simulink model "Dnote3lv3rd"  (R2016b)
settings: Solver=FixedStepDiscrete  StartTime=0.0  StopTime=simtime  RelTol=1e-3  EnableMultiTasking=on
PreLoadFcn:
  | simtime=0.0034;
undefined symbols (not defined in the file): Amp, fdesignblkfcn, Fin, Fs, FSC, gcbh, N, p, sw1, Ts
libraries: simulink x153, dspsnks4 x2, dspfdesign x1, dspvision x1, dsparch4 x1, dspmlti4 x1
(part 1 of 3)
settings Model: Creator=fumiaki  LastModifiedBy=l1tmn_main
settings Model: ModifiedComment=|
  | YUKI -- Sun Oct 02 16:05:03 2016 -- Version 1.144
  | シミュレーション前保存
settings Model: ModifiedHistory=|
  | YUKI -- Sun Oct 02 16:05:03 2016 -- Version 1.144
  | シミュレーション前保存
settings DataIOCC: LimitDataPoints=on  SaveFormat=Array  ReturnWorkspaceOutputsName=outn
settings OptimizationCC: ExpressionDepthLimit=2147483647  LifeSpan=inf
settings DebuggingCC: UnderspecifiedInitializationDetection=Classic  MergeDetectMultiDrivingBlocksExec=none  AllowSymbolicDim=off  StateNameClashWarn=warning  SFUnexpectedBacktrackingDiag=warning  SFNoUnconditionalDefaultTransitionDiag=warning  SFExecutionAtInitializationDiag=none
settings HardwareCC: ProdBitPerPointer=32  ProdBitPerSizeT=32  ProdBitPerPtrDiffT=32  ProdLargestAtomicFloat=None  ProdIntDivRoundTo=Undefined  ProdEndianess=Unspecified  ProdWordSize=32  ProdHWDeviceType=32-bit Generic
settings ModelReferenceCC: PropagateSignalLabelsOutOfModel=off
settings GRTTargetCC: TargetLangStandard=C89/C90 (ANSI)  GeneratePreprocessorConditionals=Disable all
settings ConfigComp: CovMetricSettings=dw  CovHtmlReporting=on  CovSaveCumulativeToWorkspaceVar=on  CovSaveSingleToWorkspaceVar=on  CovExternalEMLEnable=off  CovSFcnEnable=off

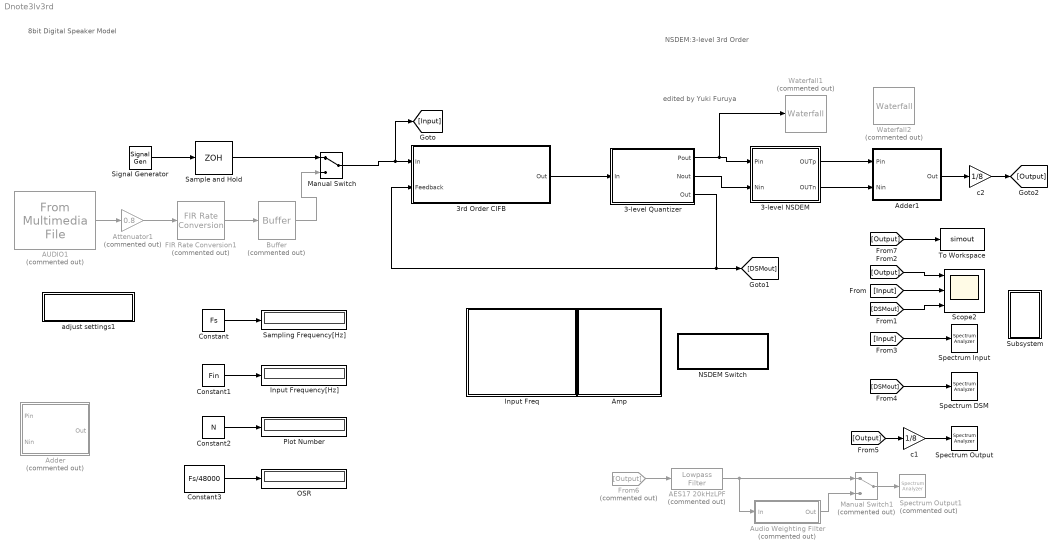
== system Dnote3lv3rd ==
  note: 8bit Digital Speaker Model
  note: edited by Yuki Furuya
  note: NSDEM:3-level 3rd Order
  "3-level NSDEM " : Subsystem  mask(3値化NSDEM){gain=[1 8 128], satulation=400}
      mask prompts: gain "フィードバック係数[1段目 2段目 ３段目]"; satulation "飽和器の値"
      mask init:
      | A=gain(1);
      | B=gain(2);
      | C=gain(3);
      | 
      | ns_fb=0;
      | 
      | SAT=satulation;
  3-level Quantizer : Subsystem
  3rd Order CIFB : Subsystem  mask(3次ΔΣ変調器(CIFB)){model=簡易モデル, FBgain=[1 3 3], INgain=[1 0 0 0], INTEGgain=[1 1 1], RESOgain=0, sat=inf}
      mask prompts: model "モデル選択"; FBgain "量子化器からのフィードバック係数 [a1 a2 a3]"; INgain "変調器から積分器の入力の係数[b1 b2 b3 b4]"; INTEGgain "積分器間の係数[c1 c2 c3]"; RESOgain "共鳴器の係数[g1]"; sat "飽和器の値[sat]"
      mask help:
      | 3次ΔΣ変調器(CIFB)のパラメータ設定
      | 簡易モデルにはa1=1; a2=3; a3=3; b1=1; b2~b4=0; c1=c2=c3=1; g1=0;を採用しています
      | 詳細モデルで任意の値を入力することが可能です。
      |
      | 係数設計にはΔΣtool boxがおすすめです。
      | 参考URL="https://pub.maruzen.co.jp/book_magazine/support/analog_digital/AppedixB_j.pdf"
      mask init:
      | if model=='簡易モデル'
      |     a1=1; a2=3; a3=3;
      |     b1=1; b2=0; b3=0; b4=0;
      |     c1=1; c2=1; c3=1;
      |     g1=0;
      |     sat=inf;
      | end
      | 
      | a1=FBgain(1);
      | a2=FBgain(2);
      | a3=FBgain(3);
      | 
      | b1=INgain(1);
      | b2=INgain(2);
      | b3=INgain(3);
      | b4=INgain(4);
      | 
      | c1=INTEGgain(1);
      | c2=INTEGgain(2);
      | c3=INTEGgain(3);
      | 
      | g1=RESOgain;
      | 
      | sat=sat;
      mask Help:
      | 3次ΔΣ変調器(CIFB)システムです。
      | 係数設定が必要です
      mask TypeOptions model: 簡易モデル | 詳細モデル
      mask Callback model:
      | enab = get_param(gcb,'model');
      | 
      | if enab=='簡易モデル'
      |     set_param(gcb,'MaskEnables',{'on','off','off','off','off','off',});
      | else
      |     set_param(gcb,'MaskEnables',{'on','on','on','on','on','on',});
      | end
  AES17 20kHzLPF : dspfdesign/Lowpass Filter  Commented=on  FilterType=FIR  DesignForMinimumOrder=on  FilterOrder=50  PassbandFrequency=20e3  StopbandFrequency=24e3  PassbandRipple=0.1  StopbandAttenuation=60  InheritSampleRate=on  SampleRate=48e3  SimulateUsing=Interpreted execution  roundingMode=Floor  coeffsDataTypeStr=fixdt(1,16)
  AUDIO1 : dspvision/From Multimedia File  Commented=on  inputFilename=/AudioSample.wav  loop=on  numPlays=1  outputStreams=Audio only  videoDataType=single  audioDataType=double  inheritSampleTime=on  userDefinedSampleTime=1/30  noAudioOutput=off  isIntensityVideo=off  fourcc=RGB  colorVideoFormat=One multidimensional signal  outputEOF=off  dataOrg=Column-major  audioFrameSize=q  computeAudioFrameSize=off  outSamplingMode=Sample based
  Adder : Subsystem  Commented=on  mask(加算器){enableerr=on, errratio=40}
      mask prompts: enableerr "製造誤差あり"; errratio "ミスマッチ[%]"
      mask help:
      | OUTpとOUTnを加算するモジュールです。
      | 誤差ありの信号が必要な場合はチェックボックスをONにしてください。
      mask init:
      | if ~enableerr
      |     err=ones(1,8);
      | else
      |     err=ones(1,8);
      |     by=errratio*0.01;
      |     a=1-by;
      |     b=1+by;
      |     rng(0,'twister');
      |     r = (b-1).*rand(1,8)+a;
      |     for i = 1:8
      |         err(i)=r(i);
      |     end
      | end
      mask Callback enableerr:
      | % Use the dialog callback to set the
      | % enabling and visibility of parameters
      | 
      | % Get the value of the Enable Bias checkbox
      | % unchecked = 'off'
      | % checked = 'on'
      | enab = get_param(gcb,'enableerr');
      | 
      | % Set the 'MaskVisililities' property for each parameters
      | if strcmp(enab,'on')
      |     set_param(gcb,'MaskVisibilities',{'on','on'});
      | else
      |     set_param(gcb,'MaskVisibilities',{'on','off'});
      | end
      | 
      | % Note that the value of the bias is not handled here.
      | % See the Initialization tab
  Adder1 : Subsystem  mask(加算器){enableerr=on, errratio=1}
      mask prompts: enableerr "製造誤差あり"; errratio "ミスマッチ[%]"
      mask help:
      | OUTpとOUTnを加算するモジュールです。
      | 誤差ありの信号が必要な場合はチェックボックスをONにしてください。
      mask init: same as Dnote3lv3rd/Adder
      mask Callback enableerr:
      | % Use the dialog callback to set the
      | % enabling and visibility of parameters
      | 
      | % Get the value of the Enable Bias checkbox
      | % unchecked = 'off'
      | % checked = 'on'
      | enab = get_param(gcb,'enableerr');
      | 
      | % Set the 'MaskVisililities' property for each parameters
      | if strcmp(enab,'on')
      |     set_param(gcb,'MaskVisibilities',{'on','on'});
      | else
      |     set_param(gcb,'MaskVisibilities',{'on','off'});
      | end
      | 
      | % Note that the value of the bias is not handled here.
      | % See the Initialization tab
  Amp : Subsystem  DialogController=hmiCreateDDGDialog  IsWebBlock=on  mask(MWDashboardBlock){webBlockId=3851c67f-551c-41d9-8c95-25d9ea438bcf, webBlockType=continuousknob, ShowInLibBrowser=on, ShowInitialText=on, HMISrcModelName=Dnote3lv3rd}
      mask prompts: webBlockId "WebBlock Id"; webBlockType "WebBlock Type"; HMISrcModelName "Source Model"
      mask Help: helpview([docroot '/mapfiles/simulink.map'], 'hmi_knob')
      mask Display:
      | if strcmp(get_param(bdroot(gcb),'BlockDiagramType'), 'library')
      |     image([(matlabroot) '/toolbox/simulink/hmi/icons/ContinuousKnob.png']);
      | end
  Attenuator1 : Gain  Commented=on  Gain=0.8  OutDataTypeStr=Inherit: Same as input  ParamDataTypeStr=Inherit: Same as input
  Audio Weighting Filter : Subsystem  Commented=on  DialogController=fdesignblkfcn  InitFcn=fdesignblkfcn(gcbh, {'InitFcn'});  mask(Audio Weighting Filter){}
      mask help: Design an audio weighting filter
      settings: CopyFcn=fdesignblkfcn(gcbh, {'CopyFcn'});
      mask Help: helpview(mapfilelocation('dsp'), 'dspaudioweightingfilter');
      mask Display: disp('Audio Weighting')
  Buffer : Buffer  Commented=on  N=1
  Constant : Constant  Value=Fs
  Constant1 : Constant  Value=Fin
  Constant2 : Constant  Value=N
  Constant3 : Constant  Value=Fs/48000
      mask Display: disp('OSR')
  FIR Rate Conversion1 : dspmlti4/FIR Rate Conversion  Commented=on  FilterSource=Dialog parameters  L=p  h=firpm(70,[0 .28 .32 1],[1 1 0 0])  M=q  FilterObject=Hm_firsrc  roundingMode=Floor  overflowMode=off  firstCoeffDataTypeStr=Inherit: Same word length as input  firstCoeffMin=[]  firstCoeffMax=[]  firstCoeffLastDataTypeStr=Inherit: Same word length as input  outputDataTypeStr=Inherit: Same as accumulator  outputMin=[]  outputMax=[]  outputLastDataTypeStr=Inherit: Same as accumulator
  From6 : From  Commented=on  GotoTag=Output
  Input Freq : Subsystem  DialogController=hmiCreateDDGDialog  IsWebBlock=on  mask(MWDashboardBlock){webBlockId=c57420c8-b641-4940-bc6c-5212ea864b9b, webBlockType=continuousknob, ShowInLibBrowser=on, ShowInitialText=on, HMISrcModelName=Dnote3lv3rd}
      mask prompts: webBlockId "WebBlock Id"; webBlockType "WebBlock Type"; HMISrcModelName "Source Model"
      mask Help: helpview([docroot '/mapfiles/simulink.map'], 'hmi_knob')
      mask Display:
      | if strcmp(get_param(bdroot(gcb),'BlockDiagramType'), 'library')
      |     image([(matlabroot) '/toolbox/simulink/hmi/icons/ContinuousKnob.png']);
      | end
  Input Frequency[Hz] : Display
  Manual Switch : ManualSwitch
  Manual Switch1 : ManualSwitch  Commented=on
  NSDEM Switch : Subsystem  DialogController=hmiCreateDDGDialog  IsWebBlock=on  mask(MathWorksWebBlock){webBlockId=b2297bbe-88b1-438d-afef-1205d982b626, webBlockType=sliderswitch, ShowInLibBrowser=on, ShowInitialText=on, HMISrcModelName=Dnote3lv3rd}
      mask prompts: webBlockId "WebBlock Id"; webBlockType "WebBlock Type"; HMISrcModelName "Source Model"
      mask Help: helpview([docroot '/mapfiles/simulink.map'], 'hmi_slider_switch')
      mask Display:
      | if strcmp(get_param(bdroot(gcb),'BlockDiagramType'), 'library')
      |     image([(matlabroot) '/toolbox/simulink/hmi/icons/SliderSwitch.png']);
      | end
  OSR : Display
  Plot Number : Display
  Sample and Hold : ZeroOrderHold  SampleTime=Ts
  Sampling Frequency[Hz] : Display
  Scope2 : Scope  NumInputPorts=3
  Signal Generator : SignalGenerator  Amplitude=Amp  Frequency=Fin
  Spectrum DSM : SpectrumAnalyzer
  Spectrum Input : SpectrumAnalyzer
  Spectrum Output : SpectrumAnalyzer
  Spectrum Output1 : SpectrumAnalyzer  Commented=on
  Subsystem : Subsystem
  To Workspace : ToWorkspace  VariableName=simout  SampleTime=-1
  Waterfall1 : dspsnks4/Waterfall  Commented=on  TraceProperties=off  NumTraces=8  CMapStr=red  TNewest=1  TOldest=0  HistoryLength=30  HistoryFull=Overwrite  UpdateInterval=1  ExportMode=Selected  MLExportName=ExportData  AutoExport=off  DisplayProperties=off  MouseMode=Orbit  AxisGrid=on  Snapshot=off  Suspend=off  SyncSnapshots=off  OpenScopeAtSimStart=off  FigPos=[657 331 413 324]  CameraView=[89.3889433100501 -276.781767245131 276.174253738902 0 5 3.5 0.767275197493131 1.68975903939443 -1.63514406758836 1.43035830301383 1 5 3]  InportDimsHint=[8 1]  AxisProperties=off  AxisColor='w'  XLabel=Speaker  YLabel=Logic  ZLabel=Time  TriggerProperties=off  TrigStartMode=Immediately  TrigStartT=0  TrigStartN=0  TrigStartFcn=trigbegin  TrigStopMode=Never  TrigStopT=0.1  TrigStopN=1  TrigStopFcn=trigend  TrigRearmMode=Never  TrigRearmT=0  TrigRearmN=0  TrigRearmFcn=trigrearm  XformProperties=on  XformMode=None  XformFcn=abs  XformExpr=(u+1)/2
      settings: YMin=0  YMax=1
  Waterfall2 : dspsnks4/Waterfall  Commented=on  TraceProperties=off  NumTraces=8  CMapStr=red  TNewest=1  TOldest=0  HistoryLength=30  HistoryFull=Overwrite  UpdateInterval=1  ExportMode=Selected  MLExportName=ExportData  AutoExport=off  DisplayProperties=off  MouseMode=Orbit  AxisGrid=on  Snapshot=off  Suspend=off  SyncSnapshots=off  OpenScopeAtSimStart=off  FigPos=[657 331 413 324]  CameraView=[89.3889433100501 -276.781767245131 276.174253738902 0 5 3.5 0.767275197493131 1.68975903939443 -1.63514406758836 1.43035830301383 1 5 3]  InportDimsHint=[8 1]  AxisProperties=off  AxisColor='w'  XLabel=Speaker  YLabel=Logic  ZLabel=Time  TriggerProperties=off  TrigStartMode=Immediately  TrigStartT=0  TrigStartN=0  TrigStartFcn=trigbegin  TrigStopMode=Never  TrigStopT=0.1  TrigStopN=1  TrigStopFcn=trigend  TrigRearmMode=Never  TrigRearmT=0  TrigRearmN=0  TrigRearmFcn=trigrearm  XformProperties=on  XformMode=None  XformFcn=abs  XformExpr=(u+1)/2
      settings: YMin=0  YMax=1
  adjust settings1 : Subsystem  Priority=1  mask(初期設定){N=48*128*50, Enablemode=on, EnableNSDEM=on, osr=128, Fin=1000, INGAIN=dBFS, Amp=0.5, AmpdB=-6}
      mask prompts: N "ポイント数(48*OSR*K, ※Kは任意の自然数)"; Enablemode "信号漏洩防止モード(推奨)"; EnableNSDEM "NSDEM使用"; osr "OSR(48kHz基準)"; Fin "入力周波数[Hz]"; INGAIN "入力振幅"; Amp "ダイヤル"; AmpdB "フルスケールに対する入力[dBFS]"
      mask help:
      | このモデルを動かすための初期設定です
      | 信号漏洩モードにチェックをいれると入力したポイント数にもっとも近い適切な値に変更してFFTを行う際に信号漏洩を防いでくれます。
      | 任意のポイント数を使用したい場合はチェックを入れないでください。
      |
      | NSDEM使用のチェックボックスはNSDEMを使用するか否かを選択することができます。
      mask init:
      | Fs=osr*48000; %サンプリング周波数
      | 
      | if EnableNSDEM
      |     sw=1;
      | else
      |     sw=0;
      | end
      | 
      | if INGAIN==1
      |     Amp=Amp;
      | else
      |     Amp=db2mag(AmpdB);
      | end
      | 
      | if Enablemode
      |      assignin('base', 'Noriginal', N);
      |     base = Fs/Fin;
      |     K = N/base;
      |     intK = round(K);
      |     N = base*intK;
      | end
      | 
      | 
      | [p,q] = rat(Fs/44100,0.0001) 
      | Ts=1/Fs;                                               %サンプリング周期
      | %fB = ceil(Fs*N/(2*osr));                   %帯域幅をfsの1/2*OSRと定義
      | %f0 = floor(2/3*fB);                            %入力信号を帯域幅内の2/3へ
      | %finrad= 2*pi/N*f0;                            %入力各周波数も正規化 to simlink
      | Offset = 1000;                                     %定常状態を扱うため初期動作の300plotは省く
      | simtime = (N+Offset)*Ts; 
      | %simtime = (N-1)*Ts; 
      | FSC=1;
      | 
      | %各変数をMATLABのワークスペースへ送る
      | assignin('base', 'simtime', simtime);
      | assignin('base','Fs' ,Fs);
      | assignin('base','Ts' ,Ts);
      | assignin('base','FSC' ,FSC);
      | assignin('base','Amp' ,Amp);
      | assignin('base','Fin' ,Fin);
      | assignin('base', 'simtime', simtime);
      | assignin('base', 'sw1', sw);
      | assignin('base', 'N', N);
      | assignin('base', 'Offset', Offset);
      | assignin('base', 'INGAIN',INGAIN );
      | assignin('base', 'p', p);
      | assignin('base', 'q', q);
      mask TypeOptions INGAIN: ダイヤル | dBFS
      mask Callback INGAIN:
      | enab = get_param(gcb,'INGAIN');
      | 
      | if enab=='ダイヤル'
      |     set_param(gcb,'MaskVisibilities',{'on','on','on','on','on','on','on','off'});
      | else
      |     set_param(gcb,'MaskVisibilities',{'on','on','on','on','on','on','off','on'});
      | end
      mask Display: disp('Simulation Settings')
  c1 : Gain  Gain=1/8  OutDataTypeStr=Inherit: Same as input  ParamDataTypeStr=Inherit: Same as input
  c2 : Gain  Gain=1/8  OutDataTypeStr=Inherit: Same as input  ParamDataTypeStr=Inherit: Same as input
  wires:
  3rd Order CIFB/1(Out) -> 3-level Quantizer/1(In)
  3-level Quantizer/3(Out) -> [DSMout], 3rd Order CIFB/2(Feedback)
  3-level Quantizer/1(Pout) -> Waterfall1/1, "3-level NSDEM "/1(Pin)
  Signal Generator/1 -> Sample and Hold/1
  AUDIO1/1 -> Attenuator1/1
  Attenuator1/1 -> FIR Rate Conversion1/1
  Sample and Hold/1 -> Manual Switch/1
  FIR Rate Conversion1/1 -> Buffer/1
  Manual Switch/1 -> [Input], 3rd Order CIFB/1(In)
  Buffer/1 -> Manual Switch/2
  Constant/1 -> Sampling Frequency[Hz]/1
  Constant1/1 -> Input Frequency[Hz]/1
  [Output] -> Scope2/1
  [Input] -> Scope2/2
  [DSMout] -> Scope2/3
  [Input] -> Spectrum Input/1
  [DSMout] -> Spectrum DSM/1
  From6/1 -> AES17 20kHzLPF/1
  Manual Switch1/1 -> Spectrum Output1/1
  AES17 20kHzLPF/1 -> Audio Weighting Filter/1(In), Manual Switch1/1
  Audio Weighting Filter/1(Out) -> Manual Switch1/2
  3-level Quantizer/2(Nout) -> "3-level NSDEM "/2(Nin)
  "3-level NSDEM "/1(OUTp) -> Adder1/1(Pin)
  "3-level NSDEM "/2(OUTn) -> Adder1/2(Nin)
  [Output] -> c1/1
  c1/1 -> Spectrum Output/1
  [Output] -> To Workspace/1
  c2/1 -> [Output]
  Adder1/1(Out) -> c2/1
  Constant2/1 -> Plot Number/1
  Constant3/1 -> OSR/1

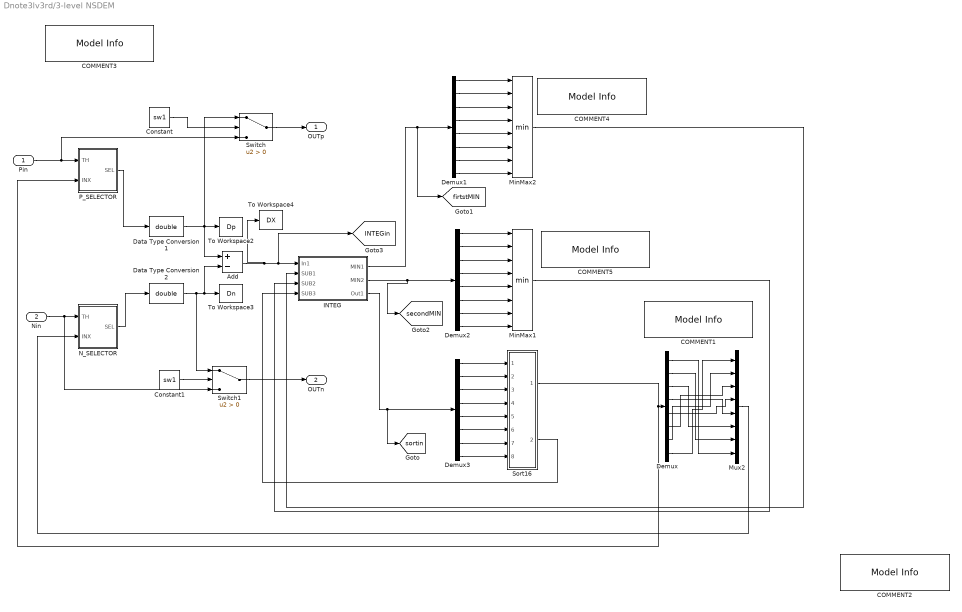
== system Dnote3lv3rd/3-level NSDEM  ==
  Pin : Inport
  Nin : Inport  Port=2
  Add : Sum  Inputs=+-
  COMMENT1 : simulink/Model-Wide Utilities/Model Info  Frame=on  DisplayStringWithTags=|  HorizontalTextAlignment=Center  LeftAlignmentValue=0.5  SourceBlockDiagram=Dnote  TagMaxNumber=20
      | バイトニックマージソートにより
      | スピーカの+側の使用頻度順に
      | 並び替え
  COMMENT2 : simulink/Model-Wide Utilities/Model Info  Frame=on  DisplayStringWithTags=p用に-側の使用頻度が少ない順に 並び替え  HorizontalTextAlignment=Center  LeftAlignmentValue=0.5  SourceBlockDiagram=Dnote  TagMaxNumber=20
  COMMENT3 : simulink/Model-Wide Utilities/Model Info  Frame=on  DisplayStringWithTags=どのスピーカを使用すべきか選択  HorizontalTextAlignment=Center  LeftAlignmentValue=0.5  SourceBlockDiagram=Dnote  TagMaxNumber=20
  COMMENT4 : simulink/Model-Wide Utilities/Model Info  Frame=on  DisplayStringWithTags=1段目の積分値の最小値  HorizontalTextAlignment=Center  LeftAlignmentValue=0.5  SourceBlockDiagram=Dnote  TagMaxNumber=20
  COMMENT5 : simulink/Model-Wide Utilities/Model Info  Frame=on  DisplayStringWithTags=2段目の積分値の最小値  HorizontalTextAlignment=Center  LeftAlignmentValue=0.5  SourceBlockDiagram=Dnote  TagMaxNumber=20
  Constant : Constant  Value=sw1
  Constant1 : Constant  Value=sw1
  Data Type Conversion1 : DataTypeConversion  OutDataTypeStr=double
  Data Type Conversion2 : DataTypeConversion  OutDataTypeStr=double
  Demux{,1..3} (4 alike) : Demux  Outputs=8
  INTEG : Subsystem
  MinMax1 : MinMax  Inputs=8
  MinMax2 : MinMax  Inputs=8
  Mux2 : Mux  Inputs=8
  N_SELECTOR : Subsystem
  P_SELECTOR : Subsystem
  Sort16 : Subsystem
  Switch : Switch  Criteria=u2 > Threshold
  Switch1 : Switch  Criteria=u2 > Threshold
  To Workspace2 : ToWorkspace  VariableName=Dp  SampleTime=-1
  To Workspace3 : ToWorkspace  VariableName=Dn  SampleTime=-1
  To Workspace4 : ToWorkspace  VariableName=DX  SampleTime=-1
  OUTp : Outport
  OUTn : Outport  Port=2
  tag scope: INTEGin=global, firtstMIN=global, secondMIN=global, sortin=global
  wires:
  Pin/1 -> Switch/3, P_SELECTOR/1(TH)
  P_SELECTOR/1(SEL) -> Data Type Conversion1/1
  Demux/8 -> Mux2/1
  Sort16/1(IDX) -> P_SELECTOR/2(INX), Demux/1
  Demux1/1 -> MinMax2/1
  Demux1/2 -> MinMax2/2
  Demux1/3 -> MinMax2/3
  Demux1/4 -> MinMax2/4
  Demux1/5 -> MinMax2/5
  Demux1/6 -> MinMax2/6
  Demux1/7 -> MinMax2/7
  Demux1/8 -> MinMax2/8
  Demux2/1 -> MinMax1/1
  Demux2/2 -> MinMax1/2
  Demux2/3 -> MinMax1/3
  Demux2/4 -> MinMax1/4
  Demux2/5 -> MinMax1/5
  Demux2/6 -> MinMax1/6
  Demux2/7 -> MinMax1/7
  Demux2/8 -> MinMax1/8
  N_SELECTOR/1(SEL) -> Data Type Conversion2/1
  Data Type Conversion1/1 -> To Workspace2/1, Switch/1, Add/1
  Add/1 -> To Workspace4/1, [INTEGin], INTEG/1(In1)
  INTEG/1(MIN1) -> [firtstMIN], Demux1/1
  INTEG/2(MIN2) -> [secondMIN], Demux2/1
  INTEG/3(Out1) -> [sortin], Demux3/1
  Demux3/1 -> Sort16/1(IN0)
  Demux3/2 -> Sort16/2(IN1)
  Demux3/3 -> Sort16/3(IN2)
  Demux3/4 -> Sort16/4(IN3)
  Demux3/5 -> Sort16/5(IN4)
  Demux3/6 -> Sort16/6(IN5)
  Demux3/7 -> Sort16/7(IN6)
  Demux3/8 -> Sort16/8(IN7)
  Sort16/2(MIN) -> INTEG/4(SUB3)
  MinMax2/1 -> INTEG/2(SUB1)
  MinMax1/1 -> INTEG/3(SUB2)
  Nin/1 -> Switch1/3, N_SELECTOR/1(TH)
  Mux2/1 -> N_SELECTOR/2(INX)
  Data Type Conversion2/1 -> Add/2, To Workspace3/1, Switch1/1
  Demux/7 -> Mux2/2
  Demux/2 -> Mux2/7
  Demux/1 -> Mux2/8
  Demux/3 -> Mux2/6
  Demux/6 -> Mux2/3
  Demux/4 -> Mux2/5
  Demux/5 -> Mux2/4
  Switch/1 -> OUTp/1
  Constant/1 -> Switch/2
  Switch1/1 -> OUTn/1
  Constant1/1 -> Switch1/2

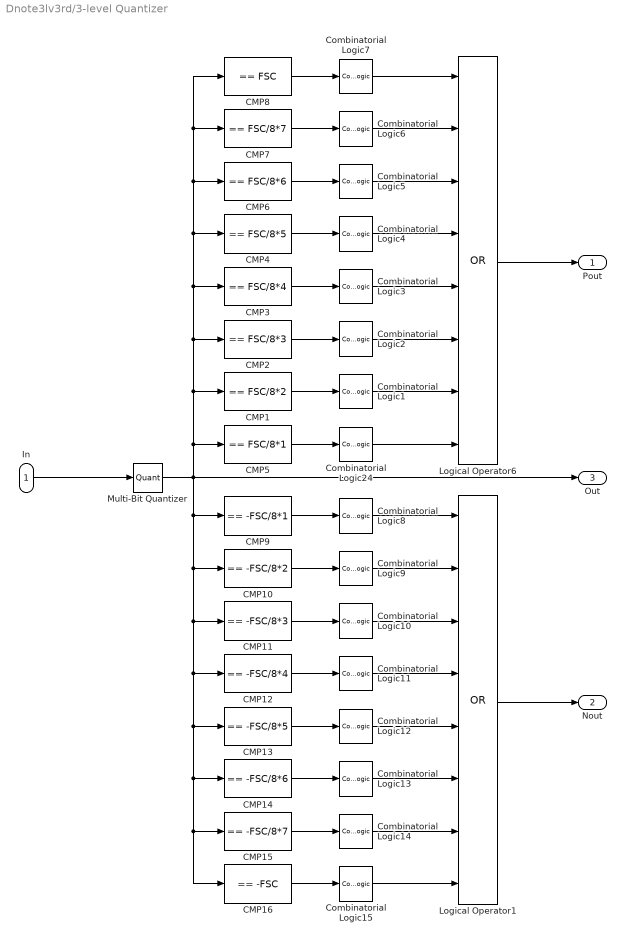
== system Dnote3lv3rd/3-level Quantizer ==
  In : Inport
  CMP1 : simulink/Logic and Bit Operations/Compare To Constant  relop===  const=FSC/8*2  OutDataTypeStr=boolean  ZeroCross=off
  CMP10 : simulink/Logic and Bit Operations/Compare To Constant  relop===  const=-FSC/8*2  OutDataTypeStr=boolean  ZeroCross=off
  CMP11 : simulink/Logic and Bit Operations/Compare To Constant  relop===  const=-FSC/8*3  OutDataTypeStr=boolean  ZeroCross=off
  CMP12 : simulink/Logic and Bit Operations/Compare To Constant  relop===  const=-FSC/8*4  OutDataTypeStr=boolean  ZeroCross=off
  CMP13 : simulink/Logic and Bit Operations/Compare To Constant  relop===  const=-FSC/8*5  OutDataTypeStr=boolean  ZeroCross=off
  CMP14 : simulink/Logic and Bit Operations/Compare To Constant  relop===  const=-FSC/8*6  OutDataTypeStr=boolean  ZeroCross=off
  CMP15 : simulink/Logic and Bit Operations/Compare To Constant  relop===  const=-FSC/8*7  OutDataTypeStr=boolean  ZeroCross=off
  CMP16 : simulink/Logic and Bit Operations/Compare To Constant  relop===  const=-FSC  OutDataTypeStr=boolean  ZeroCross=off
  CMP2 : simulink/Logic and Bit Operations/Compare To Constant  relop===  const=FSC/8*3  OutDataTypeStr=boolean  ZeroCross=off
  CMP3 : simulink/Logic and Bit Operations/Compare To Constant  relop===  const=FSC/8*4  OutDataTypeStr=boolean  ZeroCross=off
  CMP4 : simulink/Logic and Bit Operations/Compare To Constant  relop===  const=FSC/8*5  OutDataTypeStr=boolean  ZeroCross=off
  CMP5 : simulink/Logic and Bit Operations/Compare To Constant  relop===  const=FSC/8*1  OutDataTypeStr=boolean  ZeroCross=off
  CMP6 : simulink/Logic and Bit Operations/Compare To Constant  relop===  const=FSC/8*6  OutDataTypeStr=boolean  ZeroCross=off
  CMP7 : simulink/Logic and Bit Operations/Compare To Constant  relop===  const=FSC/8*7  OutDataTypeStr=boolean  ZeroCross=off
  CMP8 : simulink/Logic and Bit Operations/Compare To Constant  relop===  const=FSC  OutDataTypeStr=boolean  ZeroCross=off
  CMP9 : simulink/Logic and Bit Operations/Compare To Constant  relop===  const=-FSC/8*1  OutDataTypeStr=boolean  ZeroCross=off
  Combinatorial Logic1 : CombinatorialLogic  TruthTable=[0 0 0 0 0 0 0 0;1 1 0 0 0 0 0 0]
  Combinatorial Logic10 : CombinatorialLogic  TruthTable=[0 0 0 0 0 0 0 0;1 1 1 0 0 0 0 0]
  Combinatorial Logic11 : CombinatorialLogic  TruthTable=[0 0 0 0 0 0 0 0;1 1 1 1 0 0 0 0]
  Combinatorial Logic12 : CombinatorialLogic  TruthTable=[0 0 0 0 0 0 0 0;1 1 1 1 1 0 0 0]
  Combinatorial Logic13 : CombinatorialLogic  TruthTable=[0 0 0 0 0 0 0 0;1 1 1 1 1 1 0 0]
  Combinatorial Logic14 : CombinatorialLogic  TruthTable=[0 0 0 0 0 0 0 0;1 1 1 1 1 1 1 0]
  Combinatorial Logic15 : CombinatorialLogic  TruthTable=[0 0 0 0 0 0 0 0;1 1 1 1 1 1 1 1]
  Combinatorial Logic2 : CombinatorialLogic  TruthTable=[0 0 0 0 0 0 0 0;1 1 1 0 0 0 0 0]
  Combinatorial Logic24 : CombinatorialLogic  TruthTable=[0 0 0 0 0 0 0 0;1 0 0 0 0 0 0 0]
  Combinatorial Logic3 : CombinatorialLogic  TruthTable=[0 0 0 0 0 0 0 0;1 1 1 1 0 0 0 0]
  Combinatorial Logic4 : CombinatorialLogic  TruthTable=[0 0 0 0 0 0 0 0;1 1 1 1 1 0 0 0]
  Combinatorial Logic5 : CombinatorialLogic  TruthTable=[0 0 0 0 0 0 0 0;1 1 1 1 1 1 0 0]
  Combinatorial Logic6 : CombinatorialLogic  TruthTable=[0 0 0 0 0 0 0 0;1 1 1 1 1 1 1 0]
  Combinatorial Logic7 : CombinatorialLogic  TruthTable=[0 0 0 0 0 0 0 0;1 1 1 1 1 1 1 1]
  Combinatorial Logic8 : CombinatorialLogic  TruthTable=[0 0 0 0 0 0 0 0;1 0 0 0 0 0 0 0]
  Combinatorial Logic9 : CombinatorialLogic  TruthTable=[0 0 0 0 0 0 0 0;1 1 0 0 0 0 0 0]
  Logical Operator1 : Logic  Operator=OR  Inputs=8  AllPortsSameDT=off  OutDataTypeStr=boolean
  Logical Operator6 : Logic  Operator=OR  Inputs=8  AllPortsSameDT=off  OutDataTypeStr=boolean
  Multi-Bit Quantizer : Quantizer  QuantizationInterval=FSC/8
  Pout : Outport
  Nout : Outport  Port=2
  Out : Outport  Port=3
  wires:
  Multi-Bit Quantizer/1 -> CMP16/1, CMP15/1, CMP14/1, CMP13/1, CMP12/1, CMP11/1, CMP10/1, CMP9/1, Out/1, CMP8/1, CMP7/1, CMP6/1, CMP4/1, CMP3/1, CMP2/1, CMP1/1, CMP5/1
  Logical Operator6/1 -> Pout/1
  Logical Operator1/1 -> Nout/1
  CMP5/1 -> Combinatorial Logic24/1
  Combinatorial Logic24/1 -> Logical Operator6/8
  CMP1/1 -> Combinatorial Logic1/1
  Combinatorial Logic1/1 -> Logical Operator6/7
  CMP2/1 -> Combinatorial Logic2/1
  Combinatorial Logic2/1 -> Logical Operator6/6
  CMP3/1 -> Combinatorial Logic3/1
  Combinatorial Logic3/1 -> Logical Operator6/5
  CMP4/1 -> Combinatorial Logic4/1
  Combinatorial Logic4/1 -> Logical Operator6/4
  CMP6/1 -> Combinatorial Logic5/1
  Combinatorial Logic5/1 -> Logical Operator6/3
  CMP7/1 -> Combinatorial Logic6/1
  Combinatorial Logic6/1 -> Logical Operator6/2
  CMP8/1 -> Combinatorial Logic7/1
  Combinatorial Logic7/1 -> Logical Operator6/1
  CMP9/1 -> Combinatorial Logic8/1
  Combinatorial Logic8/1 -> Logical Operator1/1
  CMP10/1 -> Combinatorial Logic9/1
  Combinatorial Logic9/1 -> Logical Operator1/2
  CMP11/1 -> Combinatorial Logic10/1
  Combinatorial Logic10/1 -> Logical Operator1/3
  CMP12/1 -> Combinatorial Logic11/1
  Combinatorial Logic11/1 -> Logical Operator1/4
  CMP13/1 -> Combinatorial Logic12/1
  Combinatorial Logic12/1 -> Logical Operator1/5
  CMP14/1 -> Combinatorial Logic13/1
  Combinatorial Logic13/1 -> Logical Operator1/6
  CMP15/1 -> Combinatorial Logic14/1
  Combinatorial Logic14/1 -> Logical Operator1/7
  CMP16/1 -> Combinatorial Logic15/1
  Combinatorial Logic15/1 -> Logical Operator1/8
  In/1 -> Multi-Bit Quantizer/1

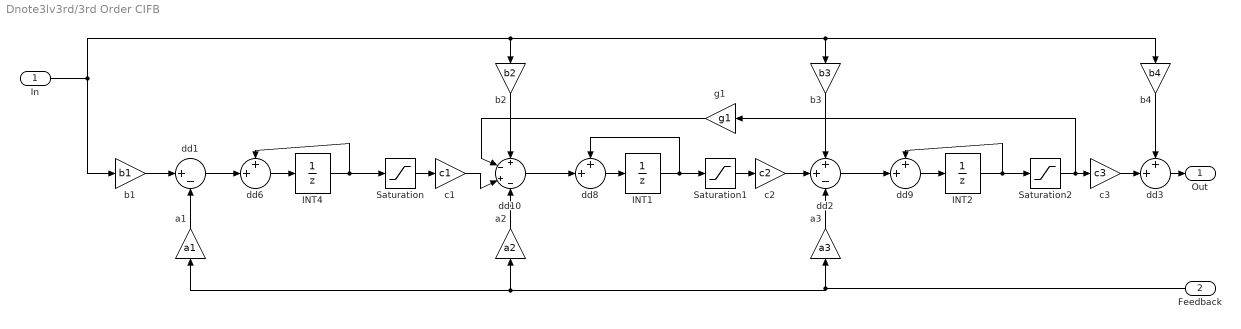
== system Dnote3lv3rd/3rd Order CIFB ==
  In : Inport
  Feedback : Inport  Port=2
  INT1 : UnitDelay  SampleTime=Ts
  INT2 : UnitDelay  SampleTime=Ts
  INT4 : UnitDelay  SampleTime=Ts
  Saturation : Saturate  UpperLimit=sat  LowerLimit=-sat
  Saturation1 : Saturate  UpperLimit=sat  LowerLimit=-sat
  Saturation2 : Saturate  UpperLimit=sat  LowerLimit=-sat
  a1 : Gain  Gain=a1  SampleTime=Ts  OutDataTypeStr=Inherit: Same as input  ParamDataTypeStr=Inherit: Same as input
  a2 : Gain  Gain=a2  SampleTime=Ts  OutDataTypeStr=Inherit: Same as input  ParamDataTypeStr=Inherit: Same as input
  a3 : Gain  Gain=a3  SampleTime=Ts  OutDataTypeStr=Inherit: Same as input  ParamDataTypeStr=Inherit: Same as input
  b1 : Gain  Gain=b1  SampleTime=Ts  SaturateOnIntegerOverflow=on  OutDataTypeStr=Inherit: Same as input  ParamDataTypeStr=Inherit: Same as input
  b2 : Gain  Gain=b2  SampleTime=Ts  SaturateOnIntegerOverflow=on  OutDataTypeStr=Inherit: Same as input  ParamDataTypeStr=Inherit: Same as input
  b3 : Gain  Gain=b3  SampleTime=Ts  SaturateOnIntegerOverflow=on  OutDataTypeStr=Inherit: Same as input  ParamDataTypeStr=Inherit: Same as input
  b4 : Gain  Gain=b4  SampleTime=Ts  SaturateOnIntegerOverflow=on  OutDataTypeStr=Inherit: Same as input  ParamDataTypeStr=Inherit: Same as input
  c1 : Gain  Gain=c1  SampleTime=Ts  OutDataTypeStr=Inherit: Same as input  ParamDataTypeStr=Inherit: Same as input
  c2 : Gain  Gain=c2  SampleTime=Ts  OutDataTypeStr=Inherit: Same as input  ParamDataTypeStr=Inherit: Same as input
  c3 : Gain  Gain=c3  SampleTime=Ts  OutDataTypeStr=Inherit: Same as input  ParamDataTypeStr=Inherit: Same as input
  dd1 : Sum  Inputs=|+-  OutDataTypeStr=double  SampleTime=Ts  SaturateOnIntegerOverflow=on  InputSameDT=on
  dd10 : Sum  Inputs=+-+-  OutDataTypeStr=double  SampleTime=Ts  SaturateOnIntegerOverflow=on  InputSameDT=on
  dd2 : Sum  Inputs=++-  OutDataTypeStr=double  SampleTime=Ts  SaturateOnIntegerOverflow=on  InputSameDT=on
  dd3 : Sum  Inputs=++|  OutDataTypeStr=double  SampleTime=Ts  SaturateOnIntegerOverflow=on  InputSameDT=on
  dd6 : Sum  Inputs=++|  OutDataTypeStr=double  SaturateOnIntegerOverflow=on  InputSameDT=on
  dd8 : Sum  Inputs=++|  OutDataTypeStr=double  SaturateOnIntegerOverflow=on  InputSameDT=on
  dd9 : Sum  Inputs=++|  OutDataTypeStr=double  SaturateOnIntegerOverflow=on  InputSameDT=on
  g1 : Gain  Gain=g1  SampleTime=Ts  SaturateOnIntegerOverflow=on  OutDataTypeStr=Inherit: Same as input  ParamDataTypeStr=Inherit: Same as input
  Out : Outport
  wires:
  dd1/1 -> dd6/2
  dd6/1 -> INT4/1
  dd8/1 -> INT1/1
  dd2/1 -> dd9/2
  dd9/1 -> INT2/1
  INT1/1 -> dd8/1, Saturation1/1
  a1/1 -> dd1/2
  INT2/1 -> dd9/1, Saturation2/1
  In/1 -> b4/1, b3/1, b2/1, b1/1
  INT4/1 -> dd6/1, Saturation/1
  Saturation/1 -> c1/1
  b1/1 -> dd1/1
  Saturation1/1 -> c2/1
  Saturation2/1 -> g1/1, c3/1
  Feedback/1 -> a2/1, a1/1, a3/1
  b2/1 -> dd10/1
  a3/1 -> dd2/3
  c2/1 -> dd2/2
  b3/1 -> dd2/1
  c3/1 -> dd3/2
  dd3/1 -> Out/1
  b4/1 -> dd3/1
  c1/1 -> dd10/3
  g1/1 -> dd10/2
  a2/1 -> dd10/4
  dd10/1 -> dd8/2

== system Dnote3lv3rd/Adder ==
  Pin : Inport
  Nin : Inport  Port=2
  Demux : Demux  Outputs=8
  Demux1 : Demux  Outputs=8
  c1 : Gain  Gain=err(1)  OutDataTypeStr=Inherit: Same as input  ParamDataTypeStr=Inherit: Same as input
  c2 : Gain  Gain=err(2)  OutDataTypeStr=Inherit: Same as input  ParamDataTypeStr=Inherit: Same as input
  c3 : Gain  Gain=err(3)  OutDataTypeStr=Inherit: Same as input  ParamDataTypeStr=Inherit: Same as input
  c4 : Gain  Gain=err(4)  OutDataTypeStr=Inherit: Same as input  ParamDataTypeStr=Inherit: Same as input
  c5 : Gain  Gain=err(5)  OutDataTypeStr=Inherit: Same as input  ParamDataTypeStr=Inherit: Same as input
  c6 : Gain  Gain=err(6)  OutDataTypeStr=Inherit: Same as input  ParamDataTypeStr=Inherit: Same as input
  c7 : Gain  Gain=err(7)  OutDataTypeStr=Inherit: Same as input  ParamDataTypeStr=Inherit: Same as input
  c8 : Gain  Gain=err(8)  OutDataTypeStr=Inherit: Same as input  ParamDataTypeStr=Inherit: Same as input
  dd{1..2,4..9} (8 alike) : Sum  Inputs=+-  OutDataTypeStr=double  SaturateOnIntegerOverflow=on  InputSameDT=on
  dd3 : Sum  Inputs=|++++++++  OutDataTypeStr=double  SaturateOnIntegerOverflow=on  InputSameDT=on
  Out : Outport
  wires:
  Pin/1 -> Demux/1
  dd3/1 -> Out/1
  Nin/1 -> Demux1/1
  Demux/1 -> dd1/1
  Demux1/8 -> dd1/2
  Demux/2 -> dd2/1
  Demux1/7 -> dd2/2
  Demux/3 -> dd4/1
  Demux1/6 -> dd4/2
  Demux/4 -> dd5/1
  Demux1/5 -> dd5/2
  Demux/5 -> dd6/1
  Demux1/4 -> dd6/2
  Demux/6 -> dd7/1
  Demux1/3 -> dd7/2
  Demux/7 -> dd9/1
  Demux1/2 -> dd9/2
  Demux/8 -> dd8/1
  Demux1/1 -> dd8/2
  dd1/1 -> c1/1
  c1/1 -> dd3/1
  dd2/1 -> c2/1
  c2/1 -> dd3/3
  dd4/1 -> c3/1
  c3/1 -> dd3/4
  dd5/1 -> c4/1
  c4/1 -> dd3/5
  dd6/1 -> c5/1
  c5/1 -> dd3/6
  dd7/1 -> c6/1
  c6/1 -> dd3/7
  dd9/1 -> c7/1
  c7/1 -> dd3/8
  dd8/1 -> c8/1
  c8/1 -> dd3/2

== system Dnote3lv3rd/Adder1 ==
  Pin : Inport
  Nin : Inport  Port=2
  Demux : Demux  Outputs=8
  Demux1 : Demux  Outputs=8
  c10 : Gain  Gain=err(6)  OutDataTypeStr=Inherit: Same as input  ParamDataTypeStr=Inherit: Same as input
  c11 : Gain  Gain=err(7)  OutDataTypeStr=Inherit: Same as input  ParamDataTypeStr=Inherit: Same as input
  c12 : Gain  Gain=err(8)  OutDataTypeStr=Inherit: Same as input  ParamDataTypeStr=Inherit: Same as input
  c13 : Gain  Gain=err(7)  OutDataTypeStr=Inherit: Same as input  ParamDataTypeStr=Inherit: Same as input
  c14 : Gain  Gain=err(8)  OutDataTypeStr=Inherit: Same as input  ParamDataTypeStr=Inherit: Same as input
  c15 : Gain  Gain=err(1)  OutDataTypeStr=Inherit: Same as input  ParamDataTypeStr=Inherit: Same as input
  c16 : Gain  Gain=err(2)  OutDataTypeStr=Inherit: Same as input  ParamDataTypeStr=Inherit: Same as input
  c17 : Gain  Gain=err(3)  OutDataTypeStr=Inherit: Same as input  ParamDataTypeStr=Inherit: Same as input
  c18 : Gain  Gain=err(4)  OutDataTypeStr=Inherit: Same as input  ParamDataTypeStr=Inherit: Same as input
  c19 : Gain  Gain=err(5)  OutDataTypeStr=Inherit: Same as input  ParamDataTypeStr=Inherit: Same as input
  c4 : Gain  Gain=err(6)  OutDataTypeStr=Inherit: Same as input  ParamDataTypeStr=Inherit: Same as input
  c5 : Gain  Gain=err(1)  OutDataTypeStr=Inherit: Same as input  ParamDataTypeStr=Inherit: Same as input
  c6 : Gain  Gain=err(2)  OutDataTypeStr=Inherit: Same as input  ParamDataTypeStr=Inherit: Same as input
  c7 : Gain  Gain=err(3)  OutDataTypeStr=Inherit: Same as input  ParamDataTypeStr=Inherit: Same as input
  c8 : Gain  Gain=err(4)  OutDataTypeStr=Inherit: Same as input  ParamDataTypeStr=Inherit: Same as input
  c9 : Gain  Gain=err(5)  OutDataTypeStr=Inherit: Same as input  ParamDataTypeStr=Inherit: Same as input
  dd3 : Sum  Inputs=|++++++++--------  OutDataTypeStr=double  SaturateOnIntegerOverflow=on  InputSameDT=on
  Out : Outport
  wires:
  c7/1 -> dd3/6
  c11/1 -> dd3/2
  Demux/2 -> c6/1
  Demux/3 -> c7/1
  Demux/6 -> c10/1
  c14/1 -> dd3/9
  c12/1 -> dd3/1
  c5/1 -> dd3/8
  c6/1 -> dd3/7
  Demux/4 -> c8/1
  c19/1 -> dd3/12
  c18/1 -> dd3/13
  c16/1 -> dd3/15
  Demux1/2 -> c16/1
  Demux/5 -> c9/1
  Demux/7 -> c11/1
  Demux/8 -> c12/1
  Demux/1 -> c5/1
  c9/1 -> dd3/4
  Demux1/3 -> c17/1
  Demux1/4 -> c18/1
  c4/1 -> dd3/11
  c10/1 -> dd3/3
  c8/1 -> dd3/5
  c13/1 -> dd3/10
  c15/1 -> dd3/16
  Demux1/6 -> c4/1
  Pin/1 -> Demux/1
  dd3/1 -> Out/1
  Demux1/7 -> c13/1
  Nin/1 -> Demux1/1
  Demux1/8 -> c14/1
  c17/1 -> dd3/14
  Demux1/1 -> c15/1
  Demux1/5 -> c19/1

== system Dnote3lv3rd/Amp ==

== system Dnote3lv3rd/Audio Weighting Filter ==
  In : Inport
  Generated Filter Block : dsparch4/Biquad Filter  Tag=BlockMethodSubSystem  IIRFiltStruct=Direct form II  CoeffSource=Specify via dialog  BiQuadCoeffs=[2.07591518974758993e-08 4.15183037949517986e-08 2.07591518974758993e-08 1 -1.97521362266648004 0.975367213791809906;1 -2 1 1 -1.99913562159154545 0.999135704628153154;1 -2 1 1 -1.99995786915622609 0.999957869599978122]  a0Flag=Warning  IC=0  ICnum=0  ICden=0  InputProcessing=Columns as channels (frame based)  denAccumFracLength=30  denProdOutputFracLength=30  secondMemoryFracLength=15  roundingMode=Floor  overflowMode=off  ScaleValues=[0.000153591125329866101;1;1;15153694.3885192499]  optimizeScaleValues=off  ScaleValueMode=Specify via input port (g)  scaleValueFracLength=14  FilterSource=Specify via dialog  FilterObject=BQF
  Out : Outport
  wires:
  In/1 -> Generated Filter Block/1
  Generated Filter Block/1 -> Out/1

== system Dnote3lv3rd/Input Freq ==

== system Dnote3lv3rd/NSDEM Switch ==

== system Dnote3lv3rd/Subsystem ==
  Demux{1..4} (4 alike) : Demux  Outputs=8
  Scope{,1..3} (4 alike) : Scope  NumInputPorts=8
  wires:
  [sortin] -> Demux3/1
  Demux3/1 -> Scope/1
  Demux3/2 -> Scope/2
  Demux3/3 -> Scope/3
  Demux3/4 -> Scope/4
  Demux3/5 -> Scope/5
  Demux3/6 -> Scope/6
  Demux3/7 -> Scope/7
  Demux3/8 -> Scope/8
  Demux1/1 -> Scope1/1
  Demux1/2 -> Scope1/2
  Demux1/3 -> Scope1/3
  Demux1/4 -> Scope1/4
  Demux1/5 -> Scope1/5
  Demux1/6 -> Scope1/6
  Demux1/7 -> Scope1/7
  Demux1/8 -> Scope1/8
  [secondMIN] -> Demux2/1
  Demux2/1 -> Scope2/1
  Demux2/2 -> Scope2/2
  Demux2/3 -> Scope2/3
  Demux2/4 -> Scope2/4
  Demux2/5 -> Scope2/5
  Demux2/6 -> Scope2/6
  Demux2/7 -> Scope2/7
  Demux2/8 -> Scope2/8
  [firtstMIN] -> Demux1/1
  [INTEGin] -> Demux4/1
  Demux4/1 -> Scope3/1
  Demux4/2 -> Scope3/2
  Demux4/3 -> Scope3/3
  Demux4/4 -> Scope3/4
  Demux4/5 -> Scope3/5
  Demux4/6 -> Scope3/6
  Demux4/7 -> Scope3/7
  Demux4/8 -> Scope3/8

== system Dnote3lv3rd/adjust settings1 ==
  note: This subsystem is empty.
      | It is used for setting parameter values (in the mask).

== system Dnote3lv3rd/3-level NSDEM /INTEG ==
  In1 : Inport
  SUB1 : Inport  Port=2
  SUB2 : Inport  Port=3
  SUB3 : Inport  Port=4
  COMMENT1 : simulink/Model-Wide Utilities/Model Info  Frame=on  DisplayStringWithTags=スピーカごとに使用回数を積分  HorizontalTextAlignment=Center  LeftAlignmentValue=0.5  SourceBlockDiagram=Dnote  TagMaxNumber=20
  COMMENT2 : simulink/Model-Wide Utilities/Model Info  Frame=on  DisplayStringWithTags=格段の積分値を引くことによって 積分値が飽和しないようにしている  HorizontalTextAlignment=Center  LeftAlignmentValue=0.5  SourceBlockDiagram=Dnote  TagMaxNumber=20
  Demux : Demux  Outputs=8
  INTEG4_1 : Subsystem
  INTEG4_2 : Subsystem
  INTEG4_3 : Subsystem
  INTEG4_4 : Subsystem
  INTEG4_5 : Subsystem
  INTEG4_6 : Subsystem
  INTEG4_7 : Subsystem
  INTEG4_8 : Subsystem
  Mux : Mux  Inputs=8
  Mux1 : Mux  Inputs=8
  Mux2 : Mux  Inputs=8
  MIN1 : Outport
  MIN2 : Outport  Port=2
  Out1 : Outport  Port=3
  wires:
  Demux/8 -> INTEG4_8/1(IN)
  Demux/7 -> INTEG4_7/1(IN)
  Demux/6 -> INTEG4_6/1(IN)
  Demux/5 -> INTEG4_5/1(IN)
  Demux/4 -> INTEG4_4/1(IN)
  Demux/3 -> INTEG4_3/1(IN)
  Demux/2 -> INTEG4_2/1(IN)
  Demux/1 -> INTEG4_1/1(IN)
  INTEG4_1/1(OUT1) -> Mux/1
  INTEG4_2/1(OUT1) -> Mux/2
  INTEG4_3/1(OUT1) -> Mux/3
  INTEG4_4/1(OUT1) -> Mux/4
  INTEG4_5/1(OUT1) -> Mux/5
  INTEG4_6/1(OUT1) -> Mux/6
  INTEG4_7/1(OUT1) -> Mux/7
  INTEG4_8/1(OUT1) -> Mux/8
  INTEG4_1/2(OUT2) -> Mux1/1
  INTEG4_2/2(OUT2) -> Mux1/2
  INTEG4_3/2(OUT2) -> Mux1/3
  INTEG4_4/2(OUT2) -> Mux1/4
  INTEG4_5/2(OUT2) -> Mux1/5
  INTEG4_6/2(OUT2) -> Mux1/6
  INTEG4_7/2(OUT2) -> Mux1/7
  INTEG4_8/2(OUT2) -> Mux1/8
  INTEG4_8/3(OUT3) -> Mux2/8
  INTEG4_7/3(OUT3) -> Mux2/7
  INTEG4_6/3(OUT3) -> Mux2/6
  INTEG4_5/3(OUT3) -> Mux2/5
  INTEG4_4/3(OUT3) -> Mux2/4
  INTEG4_3/3(OUT3) -> Mux2/3
  INTEG4_2/3(OUT3) -> Mux2/2
  INTEG4_1/3(OUT3) -> Mux2/1
  Mux/1 -> MIN1/1
  Mux1/1 -> MIN2/1
  Mux2/1 -> Out1/1
  In1/1 -> Demux/1
  SUB3/1 -> INTEG4_8/4(SUB3), INTEG4_7/4(SUB3), INTEG4_6/4(SUB3), INTEG4_5/4(SUB3), INTEG4_4/4(SUB3), INTEG4_3/4(SUB3), INTEG4_2/4(SUB3), INTEG4_1/4(SUB3)
  SUB2/1 -> INTEG4_8/3(SUB2), INTEG4_7/3(SUB2), INTEG4_6/3(SUB2), INTEG4_5/3(SUB2), INTEG4_4/3(SUB2), INTEG4_3/3(SUB2), INTEG4_2/3(SUB2), INTEG4_1/3(SUB2)
  SUB1/1 -> INTEG4_8/2(SUB1), INTEG4_7/2(SUB1), INTEG4_6/2(SUB1), INTEG4_5/2(SUB1), INTEG4_4/2(SUB1), INTEG4_3/2(SUB1), INTEG4_2/2(SUB1), INTEG4_1/2(SUB1)

== system Dnote3lv3rd/3-level NSDEM /N_SELECTOR ==
  TH : Inport
  INX : Inport  Port=2
  Constant : Constant  Value=[0 0 0 0 0 0 0 0]
  Demux : Demux  Outputs=8
  Demux1 : Demux  Outputs=8
  Logical Operator : Logic  Operator=OR  Inputs=8  AllPortsSameDT=off  OutDataTypeStr=boolean
  Subsystem : Subsystem
  Subsystem1 : Subsystem
  Subsystem2 : Subsystem
  Subsystem3 : Subsystem
  Subsystem4 : Subsystem
  Subsystem5 : Subsystem
  Subsystem6 : Subsystem
  Subsystem7 : Subsystem
  Switch{,1..7} (8 alike) : Switch  Criteria=u2 ~= 0
  SEL : Outport
  wires:
  Demux1/8 -> Switch7/2
  Demux1/7 -> Switch6/2
  Demux1/6 -> Switch5/2
  Demux1/5 -> Switch4/2
  Demux1/4 -> Switch3/2
  Demux1/3 -> Switch2/2
  Demux1/2 -> Switch1/2
  Subsystem/1(Out1) -> Switch/1
  Demux1/1 -> Switch/2
  Demux/1 -> Subsystem/1(In1)
  INX/1 -> Demux/1
  TH/1 -> Demux1/1
  Subsystem1/1(Out1) -> Switch1/1
  Subsystem2/1(Out1) -> Switch2/1
  Subsystem3/1(Out1) -> Switch3/1
  Subsystem4/1(Out1) -> Switch4/1
  Subsystem5/1(Out1) -> Switch5/1
  Subsystem6/1(Out1) -> Switch6/1
  Subsystem7/1(Out1) -> Switch7/1
  Demux/2 -> Subsystem1/1(In1)
  Demux/3 -> Subsystem2/1(In1)
  Demux/4 -> Subsystem3/1(In1)
  Demux/5 -> Subsystem4/1(In1)
  Demux/6 -> Subsystem5/1(In1)
  Demux/7 -> Subsystem6/1(In1)
  Demux/8 -> Subsystem7/1(In1)
  Switch/1 -> Logical Operator/1
  Switch1/1 -> Logical Operator/2
  Switch2/1 -> Logical Operator/3
  Switch3/1 -> Logical Operator/4
  Switch4/1 -> Logical Operator/5
  Switch5/1 -> Logical Operator/6
  Switch6/1 -> Logical Operator/7
  Switch7/1 -> Logical Operator/8
  Constant/1 -> Switch4/3, Switch/3, Switch1/3, Switch2/3, Switch3/3, Switch5/3, Switch6/3, Switch7/3
  Logical Operator/1 -> SEL/1

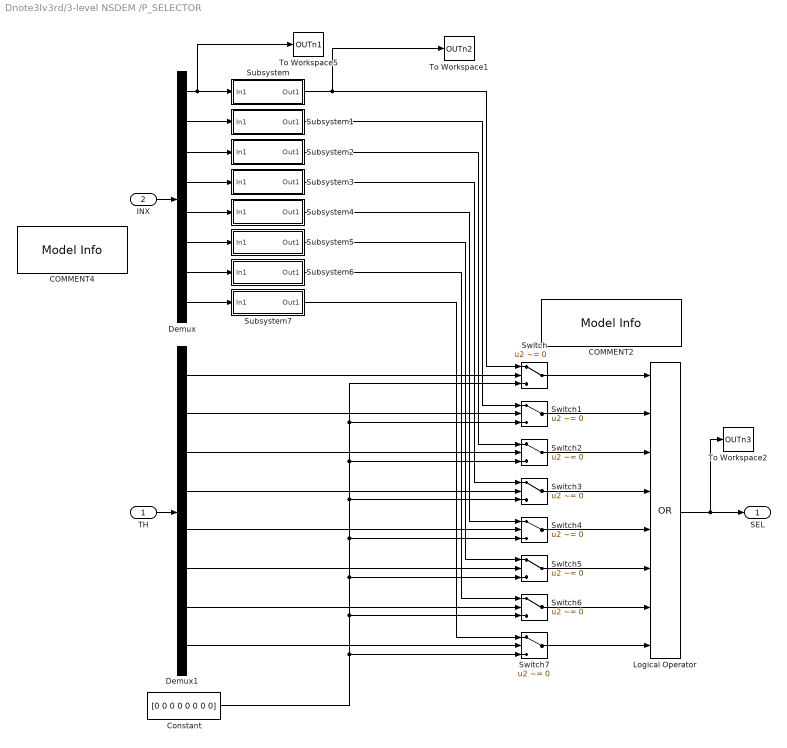
== system Dnote3lv3rd/3-level NSDEM /P_SELECTOR ==
  TH : Inport
  INX : Inport  Port=2
  COMMENT2 : simulink/Model-Wide Utilities/Model Info  Frame=on  DisplayStringWithTags=温度計コードによりスピーカの 使用個数分出力  HorizontalTextAlignment=Center  LeftAlignmentValue=0.5  SourceBlockDiagram=Dnote  TagMaxNumber=20
  COMMENT4 : simulink/Model-Wide Utilities/Model Info  Frame=on  DisplayStringWithTags=|  HorizontalTextAlignment=Center  LeftAlignmentValue=0.5  SourceBlockDiagram=Dnote  TagMaxNumber=20
      | スピーカの使用回数が少ない順に
      | 並び替えられて入力
      | 入力されるのは使用回数じゃなくどのスピーカが少ないのか
  Constant : Constant  Value=[0 0 0 0 0 0 0 0]
  Demux : Demux  Outputs=8
  Demux1 : Demux  Outputs=8
  Logical Operator : Logic  Operator=OR  Inputs=8  AllPortsSameDT=off  OutDataTypeStr=boolean
  Subsystem : Subsystem
  Subsystem1 : Subsystem
  Subsystem2 : Subsystem
  Subsystem3 : Subsystem
  Subsystem4 : Subsystem
  Subsystem5 : Subsystem
  Subsystem6 : Subsystem
  Subsystem7 : Subsystem
  Switch{,1..7} (8 alike) : Switch  Criteria=u2 ~= 0
  To Workspace1 : ToWorkspace  VariableName=OUTn2  SampleTime=-1
  To Workspace2 : ToWorkspace  VariableName=OUTn3  SampleTime=-1
  To Workspace5 : ToWorkspace  VariableName=OUTn1  SampleTime=-1
  SEL : Outport
  wires:
  Demux1/8 -> Switch7/2
  Demux1/7 -> Switch6/2
  Demux1/6 -> Switch5/2
  Demux1/5 -> Switch4/2
  Demux1/4 -> Switch3/2
  Demux1/3 -> Switch2/2
  Demux1/2 -> Switch1/2
  Subsystem/1(Out1) -> To Workspace1/1, Switch/1
  Demux1/1 -> Switch/2
  Demux/1 -> To Workspace5/1, Subsystem/1(In1)
  INX/1 -> Demux/1
  TH/1 -> Demux1/1
  Subsystem1/1(Out1) -> Switch1/1
  Subsystem2/1(Out1) -> Switch2/1
  Subsystem3/1(Out1) -> Switch3/1
  Subsystem4/1(Out1) -> Switch4/1
  Subsystem5/1(Out1) -> Switch5/1
  Subsystem6/1(Out1) -> Switch6/1
  Subsystem7/1(Out1) -> Switch7/1
  Demux/2 -> Subsystem1/1(In1)
  Demux/3 -> Subsystem2/1(In1)
  Demux/4 -> Subsystem3/1(In1)
  Demux/5 -> Subsystem4/1(In1)
  Demux/6 -> Subsystem5/1(In1)
  Demux/7 -> Subsystem6/1(In1)
  Demux/8 -> Subsystem7/1(In1)
  Switch/1 -> Logical Operator/1
  Switch1/1 -> Logical Operator/2
  Switch2/1 -> Logical Operator/3
  Switch3/1 -> Logical Operator/4
  Switch4/1 -> Logical Operator/5
  Switch5/1 -> Logical Operator/6
  Switch6/1 -> Logical Operator/7
  Switch7/1 -> Logical Operator/8
  Constant/1 -> Switch4/3, Switch/3, Switch1/3, Switch2/3, Switch3/3, Switch5/3, Switch6/3, Switch7/3
  Logical Operator/1 -> SEL/1, To Workspace2/1

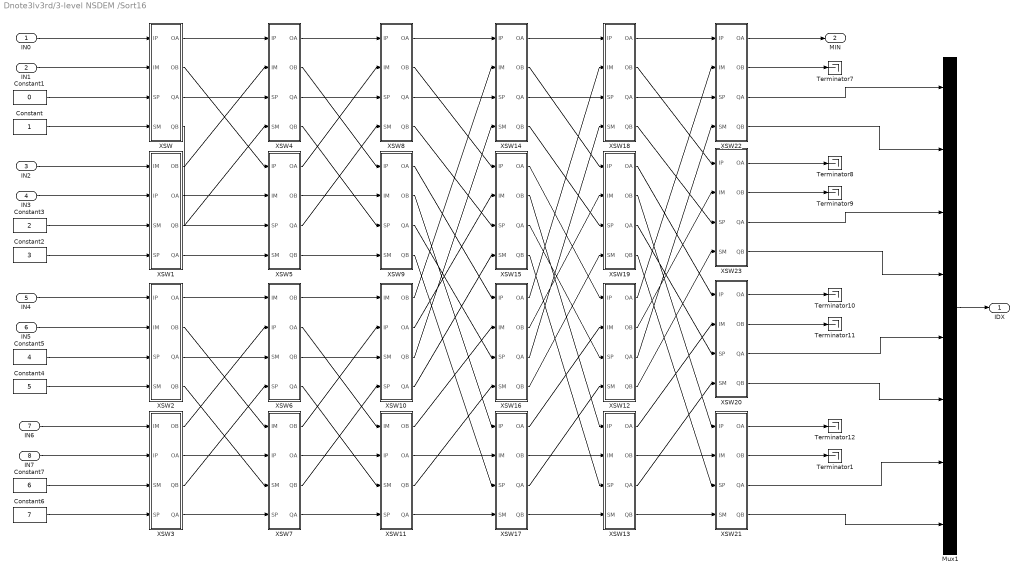
== system Dnote3lv3rd/3-level NSDEM /Sort16 ==
  IN0 : Inport
  IN1 : Inport  Port=2
  IN2 : Inport  Port=3
  IN3 : Inport  Port=4
  IN4 : Inport  Port=5
  IN5 : Inport  Port=6
  IN6 : Inport  Port=7
  IN7 : Inport  Port=8
  Constant : Constant
  Constant1 : Constant  Value=0
  Constant2 : Constant  Value=3
  Constant3 : Constant  Value=2
  Constant4 : Constant  Value=5
  Constant5 : Constant  Value=4
  Constant6 : Constant  Value=7
  Constant7 : Constant  Value=6
  Mux1 : Mux  Inputs=8
  Terminator{1,7..12} (7 alike) : Terminator
  XSW : Subsystem
  XSW1 : Subsystem
  XSW10 : Subsystem
  XSW11 : Subsystem
  XSW12 : Subsystem
  XSW13 : Subsystem
  XSW14 : Subsystem
  XSW15 : Subsystem
  XSW16 : Subsystem
  XSW17 : Subsystem
  XSW18 : Subsystem
  XSW19 : Subsystem
  XSW2 : Subsystem
  XSW20 : Subsystem
  XSW21 : Subsystem
  XSW22 : Subsystem
  XSW23 : Subsystem
  XSW3 : Subsystem
  XSW4 : Subsystem
  XSW5 : Subsystem
  XSW6 : Subsystem
  XSW7 : Subsystem
  XSW8 : Subsystem
  XSW9 : Subsystem
  IDX : Outport
  MIN : Outport  Port=2
  wires:
  XSW/1(OA) -> XSW4/1(IP)
  XSW/2(OB) -> XSW5/1(IP)
  XSW/3(QA) -> XSW4/3(SP)
  XSW/4(QB) -> XSW5/3(SP)
  XSW1/4(QA) -> XSW5/4(SM)
  XSW1/3(QB) -> XSW4/4(SM)
  XSW1/2(OA) -> XSW5/2(IM)
  XSW1/1(OB) -> XSW4/2(IM)
  XSW2/1(OA) -> XSW6/1(IM)
  XSW2/2(OB) -> XSW7/1(IM)
  XSW2/3(QA) -> XSW6/3(SM)
  XSW2/4(QB) -> XSW7/3(SM)
  XSW3/4(QA) -> XSW7/4(SP)
  XSW3/2(OA) -> XSW7/2(IP)
  XSW3/3(QB) -> XSW6/4(SP)
  XSW3/1(OB) -> XSW6/2(IP)
  XSW4/1(OA) -> XSW8/1(IP)
  XSW4/3(QA) -> XSW8/3(SP)
  XSW4/2(OB) -> XSW9/1(IP)
  XSW4/4(QB) -> XSW9/3(SP)
  XSW5/4(QB) -> XSW9/4(SM)
  XSW5/2(OB) -> XSW9/2(IM)
  XSW5/3(QA) -> XSW8/4(SM)
  XSW5/1(OA) -> XSW8/2(IM)
  XSW6/1(OB) -> XSW10/1(IM)
  XSW6/3(QB) -> XSW10/3(SM)
  XSW6/2(OA) -> XSW11/1(IM)
  XSW6/4(QA) -> XSW11/3(SM)
  XSW7/4(QA) -> XSW11/4(SP)
  XSW7/2(OA) -> XSW11/2(IP)
  XSW7/3(QB) -> XSW10/4(SP)
  XSW7/1(OB) -> XSW10/2(IP)
  XSW8/1(OA) -> XSW14/1(IP)
  XSW8/2(OB) -> XSW15/1(IP)
  XSW9/1(OA) -> XSW16/1(IP)
  XSW9/2(OB) -> XSW17/1(IP)
  XSW11/4(QA) -> XSW17/4(SM)
  XSW11/2(OA) -> XSW17/2(IM)
  XSW11/3(QB) -> XSW16/4(SM)
  XSW11/1(OB) -> XSW16/2(IM)
  XSW8/3(QA) -> XSW14/3(SP)
  XSW8/4(QB) -> XSW15/3(SP)
  XSW9/3(QA) -> XSW16/3(SP)
  XSW9/4(QB) -> XSW17/3(SP)
  XSW10/4(QA) -> XSW15/4(SM)
  XSW10/2(OA) -> XSW15/2(IM)
  XSW10/3(QB) -> XSW14/4(SM)
  XSW10/1(OB) -> XSW14/2(IM)
  XSW14/1(OA) -> XSW18/1(IP)
  XSW14/3(QA) -> XSW18/3(SP)
  XSW14/2(OB) -> XSW19/1(IP)
  XSW14/4(QB) -> XSW19/3(SP)
  XSW15/1(OA) -> XSW12/1(IP)
  XSW15/3(QA) -> XSW12/3(SP)
  XSW15/2(OB) -> XSW13/1(IP)
  XSW15/4(QB) -> XSW13/3(SP)
  XSW17/4(QB) -> XSW13/4(SM)
  XSW17/2(OB) -> XSW13/2(IM)
  XSW17/3(QA) -> XSW12/4(SM)
  XSW17/1(OA) -> XSW12/2(IM)
  XSW16/4(QB) -> XSW19/4(SM)
  XSW16/2(OB) -> XSW19/2(IM)
  XSW16/3(QA) -> XSW18/4(SM)
  XSW16/1(OA) -> XSW18/2(IM)
  XSW18/1(OA) -> XSW22/1(IP)
  XSW18/3(QA) -> XSW22/3(SP)
  XSW18/2(OB) -> XSW23/1(IP)
  XSW18/4(QB) -> XSW23/3(SP)
  XSW19/1(OA) -> XSW20/1(IP)
  XSW19/3(QA) -> XSW20/3(SP)
  XSW19/2(OB) -> XSW21/1(IP)
  XSW19/4(QB) -> XSW21/3(SP)
  XSW13/4(QB) -> XSW21/4(SM)
  XSW13/2(OB) -> XSW21/2(IM)
  XSW13/3(QA) -> XSW20/4(SM)
  XSW13/1(OA) -> XSW20/2(IM)
  XSW12/4(QB) -> XSW23/4(SM)
  XSW12/2(OB) -> XSW23/2(IM)
  XSW12/3(QA) -> XSW22/4(SM)
  XSW12/1(OA) -> XSW22/2(IM)
  XSW22/1(OA) -> MIN/1
  XSW22/2(OB) -> Terminator7/1
  XSW23/1(OA) -> Terminator8/1
  XSW23/2(OB) -> Terminator9/1
  XSW20/1(OA) -> Terminator10/1
  XSW20/2(OB) -> Terminator11/1
  XSW21/1(OA) -> Terminator12/1
  XSW21/2(OB) -> Terminator1/1
  IN0/1 -> XSW/1(IP)
  IN1/1 -> XSW/2(IM)
  Constant1/1 -> XSW/3(SP)
  Constant/1 -> XSW/4(SM)
  IN2/1 -> XSW1/1(IM)
  IN3/1 -> XSW1/2(IP)
  Constant3/1 -> XSW1/3(SM)
  Constant2/1 -> XSW1/4(SP)
  IN4/1 -> XSW2/1(IP)
  IN5/1 -> XSW2/2(IM)
  Constant5/1 -> XSW2/3(SP)
  Constant4/1 -> XSW2/4(SM)
  IN6/1 -> XSW3/1(IM)
  IN7/1 -> XSW3/2(IP)
  Constant7/1 -> XSW3/3(SM)
  Constant6/1 -> XSW3/4(SP)
  XSW21/4(QB) -> Mux1/8
  XSW21/3(QA) -> Mux1/7
  Mux1/1 -> IDX/1
  XSW20/4(QB) -> Mux1/6
  XSW20/3(QA) -> Mux1/5
  XSW22/3(QA) -> Mux1/1
  XSW22/4(QB) -> Mux1/2
  XSW23/3(QA) -> Mux1/3
  XSW23/4(QB) -> Mux1/4

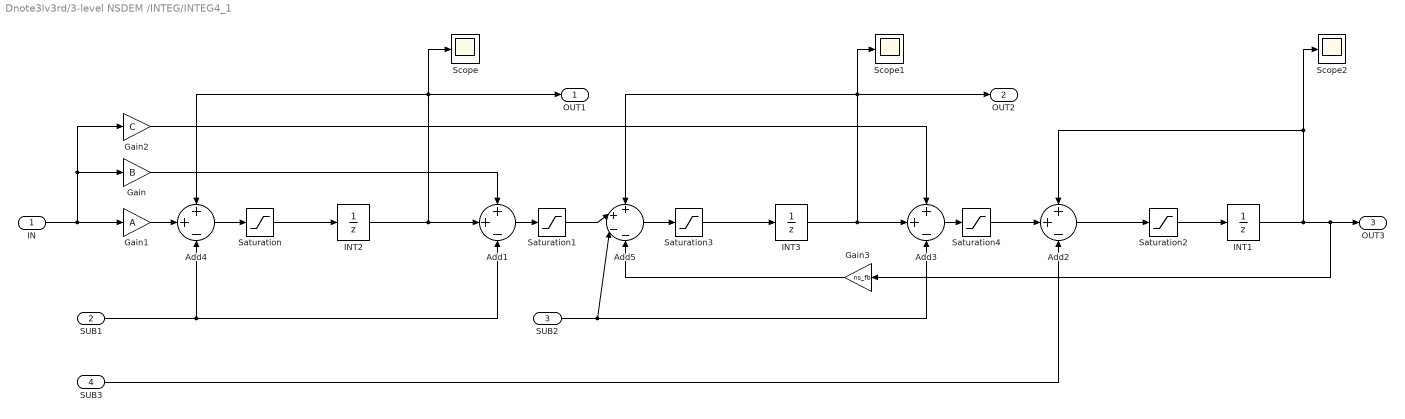
== system Dnote3lv3rd/3-level NSDEM /INTEG/INTEG4_1 ==
  IN : Inport
  SUB1 : Inport  Port=2
  SUB2 : Inport  Port=3
  SUB3 : Inport  Port=4
  Add{1..4} (4 alike) : Sum  Inputs=++-
  Add5 : Sum  Inputs=++--
  Gain : Gain  Gain=B
  Gain1 : Gain  Gain=A
  Gain2 : Gain  Gain=C
  Gain3 : Gain  Gain=ns_fb
  INT1 : UnitDelay  SampleTime=Ts
  INT2 : UnitDelay  SampleTime=Ts
  INT3 : UnitDelay  SampleTime=Ts
  Saturation{,1..4} (5 alike) : Saturate  UpperLimit=SAT  LowerLimit=-SAT
  Scope : Scope
  Scope1 : Scope
  Scope2 : Scope
  OUT1 : Outport
  OUT2 : Outport  Port=2
  OUT3 : Outport  Port=3
  wires:
  Gain1/1 -> Add4/2
  Saturation1/1 -> Add5/2
  Saturation4/1 -> Add2/2
  Gain2/1 -> Add3/1
  Add3/1 -> Saturation4/1
  SUB2/1 -> Add3/3, Add5/3
  Add5/1 -> Saturation3/1
  Add2/1 -> Saturation2/1
  Gain/1 -> Add1/1
  Add1/1 -> Saturation1/1
  IN/1 -> Gain1/1, Gain2/1, Gain/1
  SUB1/1 -> Add4/3, Add1/3
  Add4/1 -> Saturation/1
  SUB3/1 -> Add2/3
  Gain3/1 -> Add5/4
  INT1/1 -> Scope2/1, Add2/1, Gain3/1, OUT3/1
  INT3/1 -> Add3/2, Scope1/1, OUT2/1, Add5/1
  Saturation2/1 -> INT1/1
  INT2/1 -> Scope/1, OUT1/1, Add4/1, Add1/2
  Saturation/1 -> INT2/1
  Saturation3/1 -> INT3/1

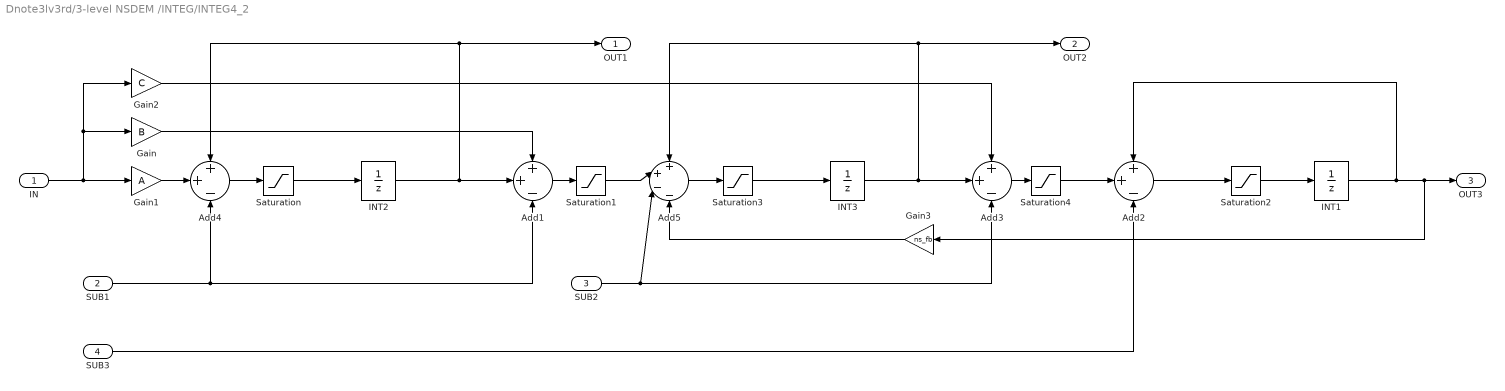
== system Dnote3lv3rd/3-level NSDEM /INTEG/INTEG4_2 ==
  IN : Inport
  SUB1 : Inport  Port=2
  SUB2 : Inport  Port=3
  SUB3 : Inport  Port=4
  Add{1..4} (4 alike) : Sum  Inputs=++-
  Add5 : Sum  Inputs=++--
  Gain : Gain  Gain=B
  Gain1 : Gain  Gain=A
  Gain2 : Gain  Gain=C
  Gain3 : Gain  Gain=ns_fb
  INT1 : UnitDelay  SampleTime=Ts
  INT2 : UnitDelay  SampleTime=Ts
  INT3 : UnitDelay  SampleTime=Ts
  Saturation{,1..4} (5 alike) : Saturate  UpperLimit=SAT  LowerLimit=-SAT
  OUT1 : Outport
  OUT2 : Outport  Port=2
  OUT3 : Outport  Port=3
  wires:
  Gain1/1 -> Add4/2
  Saturation1/1 -> Add5/2
  Saturation4/1 -> Add2/2
  Gain2/1 -> Add3/1
  Add3/1 -> Saturation4/1
  SUB2/1 -> Add3/3, Add5/3
  Add5/1 -> Saturation3/1
  Add2/1 -> Saturation2/1
  Gain/1 -> Add1/1
  Add1/1 -> Saturation1/1
  IN/1 -> Gain1/1, Gain2/1, Gain/1
  SUB1/1 -> Add4/3, Add1/3
  Add4/1 -> Saturation/1
  SUB3/1 -> Add2/3
  Gain3/1 -> Add5/4
  INT1/1 -> Add2/1, Gain3/1, OUT3/1
  INT3/1 -> Add3/2, OUT2/1, Add5/1
  Saturation2/1 -> INT1/1
  INT2/1 -> OUT1/1, Add4/1, Add1/2
  Saturation/1 -> INT2/1
  Saturation3/1 -> INT3/1

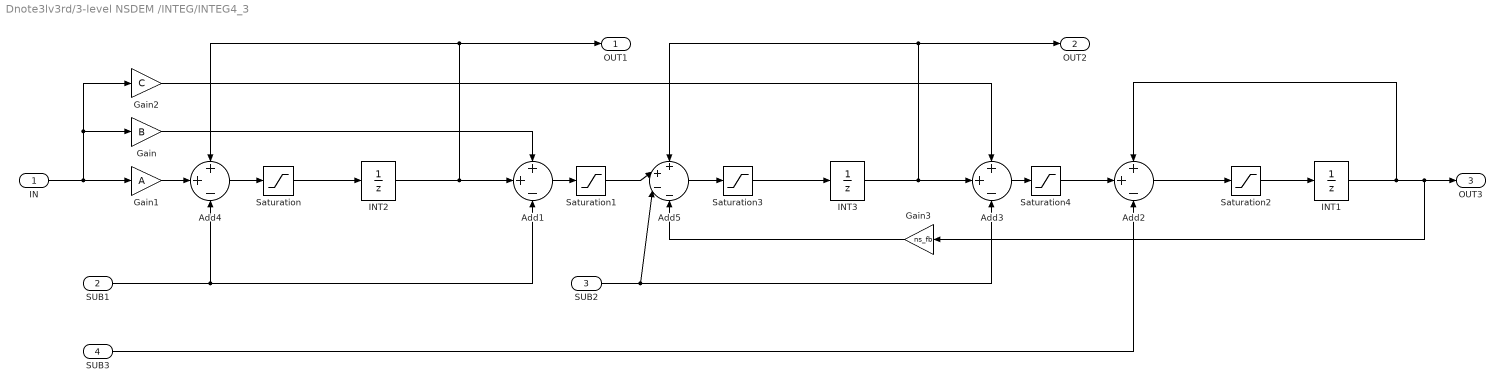
== system Dnote3lv3rd/3-level NSDEM /INTEG/INTEG4_3 ==
  IN : Inport
  SUB1 : Inport  Port=2
  SUB2 : Inport  Port=3
  SUB3 : Inport  Port=4
  Add{1..4} (4 alike) : Sum  Inputs=++-
  Add5 : Sum  Inputs=++--
  Gain : Gain  Gain=B
  Gain1 : Gain  Gain=A
  Gain2 : Gain  Gain=C
  Gain3 : Gain  Gain=ns_fb
  INT1 : UnitDelay  SampleTime=Ts
  INT2 : UnitDelay  SampleTime=Ts
  INT3 : UnitDelay  SampleTime=Ts
  Saturation{,1..4} (5 alike) : Saturate  UpperLimit=SAT  LowerLimit=-SAT
  OUT1 : Outport
  OUT2 : Outport  Port=2
  OUT3 : Outport  Port=3
  wires:
  Gain1/1 -> Add4/2
  Saturation1/1 -> Add5/2
  Saturation4/1 -> Add2/2
  Gain2/1 -> Add3/1
  Add3/1 -> Saturation4/1
  SUB2/1 -> Add3/3, Add5/3
  Add5/1 -> Saturation3/1
  Add2/1 -> Saturation2/1
  Gain/1 -> Add1/1
  Add1/1 -> Saturation1/1
  IN/1 -> Gain1/1, Gain2/1, Gain/1
  SUB1/1 -> Add4/3, Add1/3
  Add4/1 -> Saturation/1
  SUB3/1 -> Add2/3
  Gain3/1 -> Add5/4
  INT1/1 -> Add2/1, Gain3/1, OUT3/1
  INT3/1 -> Add3/2, OUT2/1, Add5/1
  Saturation2/1 -> INT1/1
  INT2/1 -> OUT1/1, Add4/1, Add1/2
  Saturation/1 -> INT2/1
  Saturation3/1 -> INT3/1

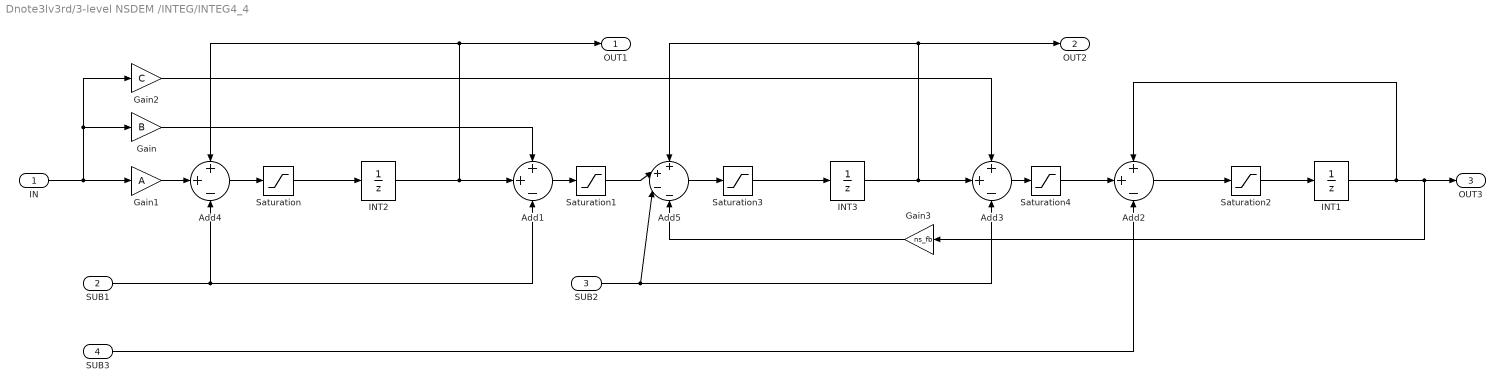
== system Dnote3lv3rd/3-level NSDEM /INTEG/INTEG4_4 ==
  IN : Inport
  SUB1 : Inport  Port=2
  SUB2 : Inport  Port=3
  SUB3 : Inport  Port=4
  Add{1..4} (4 alike) : Sum  Inputs=++-
  Add5 : Sum  Inputs=++--
  Gain : Gain  Gain=B
  Gain1 : Gain  Gain=A
  Gain2 : Gain  Gain=C
  Gain3 : Gain  Gain=ns_fb
  INT1 : UnitDelay  SampleTime=Ts
  INT2 : UnitDelay  SampleTime=Ts
  INT3 : UnitDelay  SampleTime=Ts
  Saturation{,1..4} (5 alike) : Saturate  UpperLimit=SAT  LowerLimit=-SAT
  OUT1 : Outport
  OUT2 : Outport  Port=2
  OUT3 : Outport  Port=3
  wires:
  Gain1/1 -> Add4/2
  Saturation1/1 -> Add5/2
  Saturation4/1 -> Add2/2
  Gain2/1 -> Add3/1
  Add3/1 -> Saturation4/1
  SUB2/1 -> Add3/3, Add5/3
  Add5/1 -> Saturation3/1
  Add2/1 -> Saturation2/1
  Gain/1 -> Add1/1
  Add1/1 -> Saturation1/1
  IN/1 -> Gain1/1, Gain2/1, Gain/1
  SUB1/1 -> Add4/3, Add1/3
  Add4/1 -> Saturation/1
  SUB3/1 -> Add2/3
  Gain3/1 -> Add5/4
  INT1/1 -> Add2/1, Gain3/1, OUT3/1
  INT3/1 -> Add3/2, OUT2/1, Add5/1
  Saturation2/1 -> INT1/1
  INT2/1 -> OUT1/1, Add4/1, Add1/2
  Saturation/1 -> INT2/1
  Saturation3/1 -> INT3/1
